simulink model "robot005"  (R2016a)
settings: Solver=FixedStepDiscrete  StartTime=0.0  StopTime=inf  FixedStep=0.001  RelTol=1e-3
libraries: SIA_Robot_Toolbox x9
settings Model: SimulationMode=external  Creator=Administrator  LastModifiedBy=HP
settings OptimizationCC: OptimizeModelRefInitCode=on  LifeSpan=Inf
settings RTWCC: SystemTargetFile=linux_ert_target.tlc  GenCodeOnly=on  MakeCommand=make_rtw CC=gcc  TemplateMakefile=linux_ert_target.tmf  Description=Linux Embedded Real-Time target  RetainRTWFile=on
settings CodeAppCC: ForceParamTrailComments=on  IgnoreCustomStorageClasses=off  OperatorAnnotations=on  SimulinkDataObjDesc=on  SFDataObjDesc=on  MATLABFcnDesc=on  InsertBlockDesc=on  MATLABSourceComments=on
settings STFCustomTargetCC: CombineOutputUpdateFcns=on  ERTCustomFileBanners=on  SupportNonInlinedSFcns=off  MATLABClassNameForMDSCustomization=Simulink.SoftwareTarget.ERTCustomization  GRTInterface=off  SystemTargetFile=linux_ert_target.tlc
settings ERTTargetCC: ParMdlRefBuildCompliant=off  CompOptLevelCompliant=off  ConcurrentExecutionCompliant=off  SupportContinuousTime=on  ModelStepFunctionPrototypeControlCompliant=off  CPPClassGenCompliant=off  UseToolchainInfoCompliant=off  ExtMode=on  ExtModeMexArgs='192.168.0.99' 1 17725  ERTSrcFileBannerTemplate=linux_ert_target_code_template.cgt  ERTHdrFileBannerTemplate=linux_ert_target_code_template.cgt  ERTDataSrcFileTemplate=linux_ert_target_code_template.cgt  ERTDataHdrFileTemplate=linux_ert_target_code_template.cgt  ERTCustomFileTemplate=linux_ert_target_generate_main.tlc
settings SimscapeCC: SimscapeNormalizeSystem=off

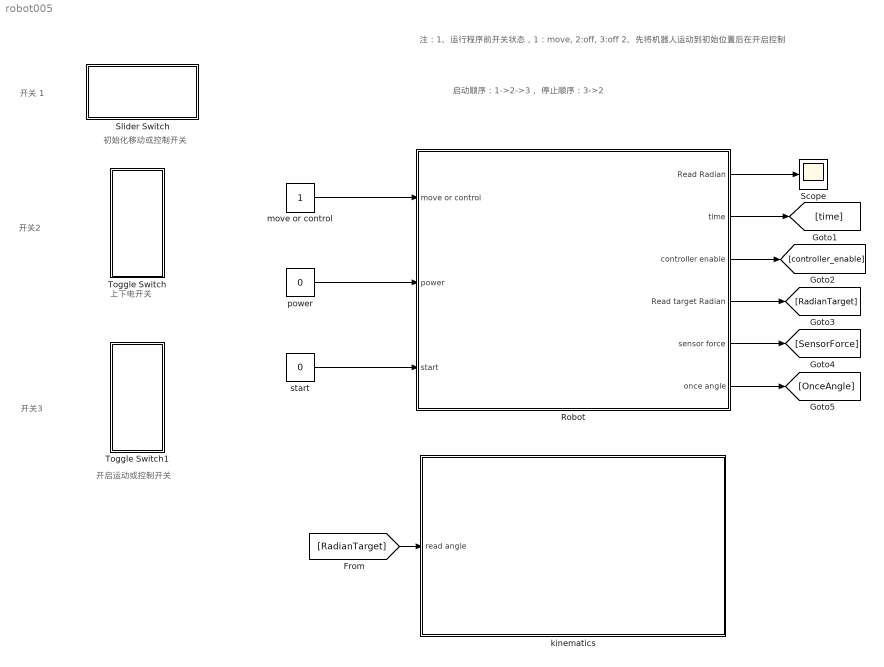
== system robot005 ==
  note: 启动顺序：1->2->3，
      | 停止顺序：3->2
  note: 开关 1
  note: 注：1、运行程序前开关状态，1：move, 2:off, 3:off
      | 2、先将机器人运动到初始位置后在开启控制
  note: 开启运动或控制开关
  note: 上下电开关
  note: 初始化移动或控制开关
  note: 开关2
  note: 开关3
  Robot : Subsystem  mask(模块说明){move_joint=[1 0.6 0 0 1 0]}
      mask prompts: move_joint "move_joint(rad)"
      mask help: 不需要更改该模块内部程序。
  Scope : Scope
  Slider Switch : Subsystem  DialogController=hmiCreateDDGDialog  IsWebBlock=on  mask(MWDashboardBlock){webBlockId=e487defa-cf66-408f-93df-043974d5a550, webBlockType=sliderswitch, ShowInLibBrowser=on, ShowInitialText=on, HMISrcModelName=robot005_2016a}
      mask prompts: webBlockId "WebBlock Id"; webBlockType "WebBlock Type"; HMISrcModelName "Source Model"
      mask help: Set on/off value to tune parameters or variables.
      mask Help: helpview([docroot '/mapfiles/simulink.map'], 'hmi_switch')
      mask Display:
      | if strcmp(get_param(bdroot(gcb),'BlockDiagramType'),'library')
      |  image([(matlabroot) '/toolbox/simulink/hmi/icons/SliderSwitch.png'])
      | end
  Toggle Switch : Subsystem  DialogController=hmiCreateDDGDialog  IsWebBlock=on  mask(MWDashboardBlock){webBlockId=df158d09-57bd-48b0-a65e-f3d7cce1d0b3, webBlockType=toggleswitch, ShowInLibBrowser=on, ShowInitialText=on, HMISrcModelName=robot005_2016a}
      mask prompts: webBlockId "WebBlock Id"; webBlockType "WebBlock Type"; HMISrcModelName "Source Model"
      mask help: Set on/off value to tune parameters or variables.
      mask Help: helpview([docroot '/mapfiles/simulink.map'], 'hmi_switch')
      mask Display:
      | if strcmp(get_param(bdroot(gcb),'BlockDiagramType'),'library')
      |  image([(matlabroot) '/toolbox/simulink/hmi/icons/ToggleSwitch.png'])
      | end
  Toggle Switch1 : Subsystem  DialogController=hmiCreateDDGDialog  IsWebBlock=on  mask(MWDashboardBlock){webBlockId=392d6191-f6a5-4e6d-a801-0994c69ad5e5, webBlockType=toggleswitch, ShowInLibBrowser=on, ShowInitialText=on, HMISrcModelName=robot005_2016a}
      mask prompts: webBlockId "WebBlock Id"; webBlockType "WebBlock Type"; HMISrcModelName "Source Model"
      mask help: Set on/off value to tune parameters or variables.
      mask Help: helpview([docroot '/mapfiles/simulink.map'], 'hmi_switch')
      mask Display:
      | if strcmp(get_param(bdroot(gcb),'BlockDiagramType'),'library')
      |  image([(matlabroot) '/toolbox/simulink/hmi/icons/ToggleSwitch.png'])
      | end
  kinematics : Subsystem
  move or control : Constant
  power : Constant  Value=0
  start : Constant  Value=0
  wires:
  move or control/1 -> Robot/1(move or control)
  power/1 -> Robot/2(power)
  Robot/1(Read Radian) -> Scope/1
  Robot/2(time) -> [time]
  Robot/3(controller enable) -> [controller_enable]
  Robot/4(Read target Radian) -> [RadianTarget]
  Robot/5(sensor force) -> [SensorForce]
  Robot/6(once angle) -> [OnceAngle]
  start/1 -> Robot/3(start)
  [RadianTarget] -> kinematics/1(read angle)

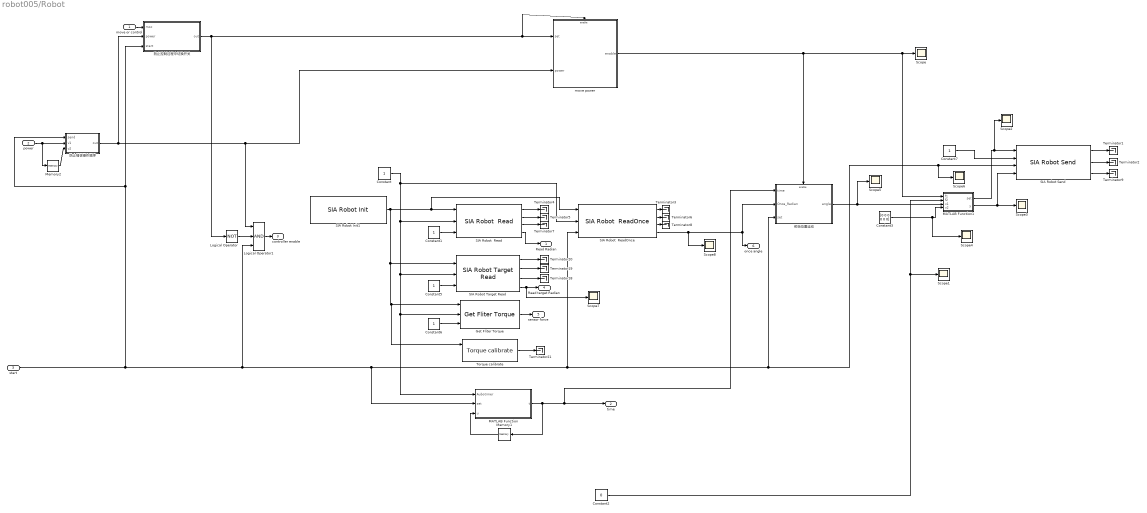
== system robot005/Robot ==
  move or control : Inport
  power : Inport  Port=2
  start : Inport  Port=3
  " Torque calibrate" : SIA_Robot_Toolbox/Sensor/ Torque calibrate
  Constant{,1,5..7} (5 alike) : Constant
  Constant2 : Constant  Value=0
  Constant3 : Constant  Value=[0 0 0 0 0 0]
  Get Fliter Torque : SIA_Robot_Toolbox/Sensor/Get Fliter Torque  p_buf_num_sensor=20
  Logical Operator : Logic  Operator=NOT  AllPortsSameDT=off  OutDataTypeStr=boolean
  Logical Operator1 : Logic  Inputs=3  AllPortsSameDT=off  OutDataTypeStr=boolean
  MATLAB Function : MATLAB Function  TreatAsAtomicUnit=on
  MATLAB Function1 : MATLAB Function  TreatAsAtomicUnit=on
  Memory1 : Memory
  Memory2 : Memory
  SIA Robot  Read : SIA_Robot_Toolbox/Robot Interface/SIA Robot  Read  g_Axisnum=6
  SIA Robot  ReadOnce : SIA_Robot_Toolbox/Robot Interface/SIA Robot  ReadOnce  g_Axisnum=6
  SIA Robot Init1 : SIA_Robot_Toolbox/Robot System Tool/SIA Robot Init  p_AUBO=on
  SIA Robot Send : SIA_Robot_Toolbox/Robot Interface/SIA Robot Send  g_Axisnum=6
  SIA Robot Target Read : SIA_Robot_Toolbox/Robot Interface/SIA Robot Target Read
  Scope{,1..8} (9 alike) : Scope
  Terminator{1..9,18..21} (13 alike) : Terminator
  move power : Subsystem
  初始位置运动 : Subsystem
  防止控制过程中切换开关 : MATLAB Function  TreatAsAtomicUnit=on
  防止错误操作顺序 : MATLAB Function  TreatAsAtomicUnit=on
  Read Radian : Outport
  time : Outport  Port=2
  controller enable : Outport  Port=3
  Read target Radian : Outport  Port=4
  sensor force : Outport  Port=5
  once angle : Outport  Port=6
  wires:
  Constant/1 -> SIA Robot  ReadOnce/2, SIA Robot  Read/2, SIA Robot Target Read/2, MATLAB Function/1(Aubotimer), Get Fliter Torque/2
  SIA Robot Init1/1 -> " Torque calibrate"/1, Get Fliter Torque/1, SIA Robot Target Read/1, SIA Robot  ReadOnce/1, SIA Robot  Read/1
  Constant1/1 -> SIA Robot  Read/3
  Memory1/1 -> MATLAB Function/3(u)
  SIA Robot Send/1 -> Terminator1/1
  SIA Robot Send/2 -> Terminator2/1
  SIA Robot  ReadOnce/1 -> Terminator3/1
  SIA Robot  Read/4 -> Read Radian/1
  SIA Robot  ReadOnce/4 -> Scope8/1, 初始位置运动/2(Once_Radian), once angle/1
  MATLAB Function/1(t) -> 初始位置运动/1(time), time/1, Memory1/1
  start/1 -> 防止控制过程中切换开关/3(start), 防止错误操作顺序/1(send), Logical Operator1/3, MATLAB Function/2(set), SIA Robot  ReadOnce/3, 初始位置运动/3(set), Scope6/1, SIA Robot Send/3
  SIA Robot  Read/1 -> Terminator4/1
  SIA Robot  Read/2 -> Terminator5/1
  SIA Robot  ReadOnce/2 -> Terminator6/1
  SIA Robot  Read/3 -> Terminator7/1
  SIA Robot  ReadOnce/3 -> Terminator8/1
  SIA Robot Send/3 -> Terminator9/1
  初始位置运动/1(angle) -> MATLAB Function1/3(v1), Scope5/1
  防止错误操作顺序/1(out) -> 防止控制过程中切换开关/2(power), Logical Operator1/1, move power/2(power)
  防止控制过程中切换开关/1(out) -> Logical Operator/1, move power/Enable, move power/1(set)
  move or control/1 -> 防止控制过程中切换开关/1(moc)
  Memory2/1 -> 防止错误操作顺序/3(v2)
  power/1 -> Memory2/1, 防止错误操作顺序/2(v1)
  Logical Operator1/1 -> controller enable/1
  Logical Operator/1 -> Logical Operator1/2
  Constant5/1 -> SIA Robot Target Read/3
  SIA Robot Target Read/4 -> Scope7/1, Read target Radian/1
  SIA Robot Target Read/3 -> Terminator18/1
  SIA Robot Target Read/2 -> Terminator19/1
  SIA Robot Target Read/1 -> Terminator20/1
  Constant6/1 -> Get Fliter Torque/3
  Get Fliter Torque/1 -> sensor force/1
  " Torque calibrate"/1 -> Terminator21/1
  Constant7/1 -> SIA Robot Send/2
  MATLAB Function1/1(set) -> Scope2/1, SIA Robot Send/1
  Constant3/1 -> Scope4/1, MATLAB Function1/4(v2)
  MATLAB Function1/2(y) -> Scope3/1, SIA Robot Send/4
  move power/1(enable) -> 初始位置运动/Enable, MATLAB Function1/1(f1), Scope/1
  Constant2/1 -> MATLAB Function1/2(f2), Scope1/1

== system robot005/Slider Switch ==

== system robot005/Toggle Switch ==

== system robot005/Toggle Switch1 ==

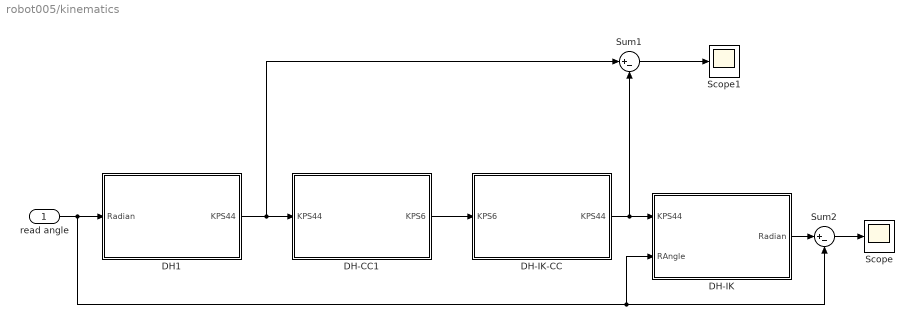
== system robot005/kinematics ==
  read angle : Inport
  DH-CC1 : MATLAB Function  TreatAsAtomicUnit=on
  DH-IK : MATLAB Function  TreatAsAtomicUnit=on
  DH-IK-CC : MATLAB Function  TreatAsAtomicUnit=on
  DH1 : MATLAB Function  TreatAsAtomicUnit=on
  Scope : Scope
  Scope1 : Scope
  Sum1 : Sum  Inputs=|+-
  Sum2 : Sum  Inputs=|+-
  wires:
  DH1/1(KPS44) -> DH-CC1/1(KPS44), Sum1/1
  read angle/1 -> DH1/1(Radian), DH-IK/2(RAngle), Sum2/2
  DH-CC1/1(KPS6) -> DH-IK-CC/1(KPS6)
  DH-IK-CC/1(KPS44) -> DH-IK/1(KPS44), Sum1/2
  DH-IK/1(Radian) -> Sum2/1
  Sum2/1 -> Scope/1
  Sum1/1 -> Scope1/1

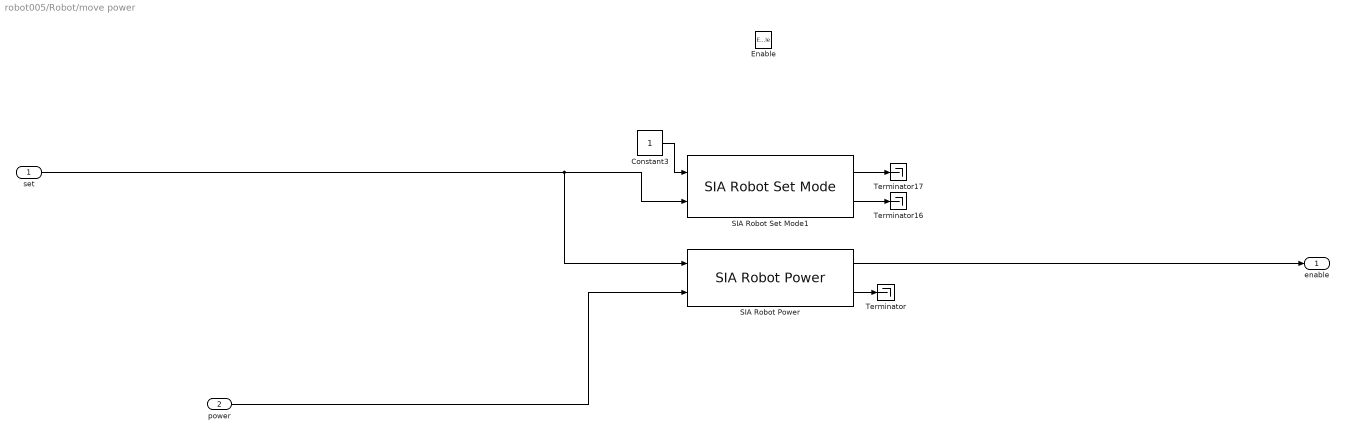
== system robot005/Robot/move power ==
  set : Inport
  power : Inport  Port=2
  Enable : EnablePort
  Constant3 : Constant
  SIA Robot Power : SIA_Robot_Toolbox/Robot System Tool/SIA Robot Power
  SIA Robot Set Mode1 : SIA_Robot_Toolbox/Robot Interface/SIA Robot Set Mode  Axis_1=off  Axis_2=off  Axis_3=off  Axis_4=off  Axis_5=off  Axis_6=off
      link override S-Function Builder: Parameters=Axis_1,Axis_2,Axis_3,Axis_4,Axis_5,Axis_6
  Terminator : Terminator
  Terminator16 : Terminator
  Terminator17 : Terminator
  enable : Outport
  wires:
  power/1 -> SIA Robot Power/2
  set/1 -> SIA Robot Power/1, SIA Robot Set Mode1/2
  SIA Robot Power/2 -> Terminator/1
  Constant3/1 -> SIA Robot Set Mode1/1
  SIA Robot Power/1 -> enable/1
  SIA Robot Set Mode1/2 -> Terminator16/1
  SIA Robot Set Mode1/1 -> Terminator17/1

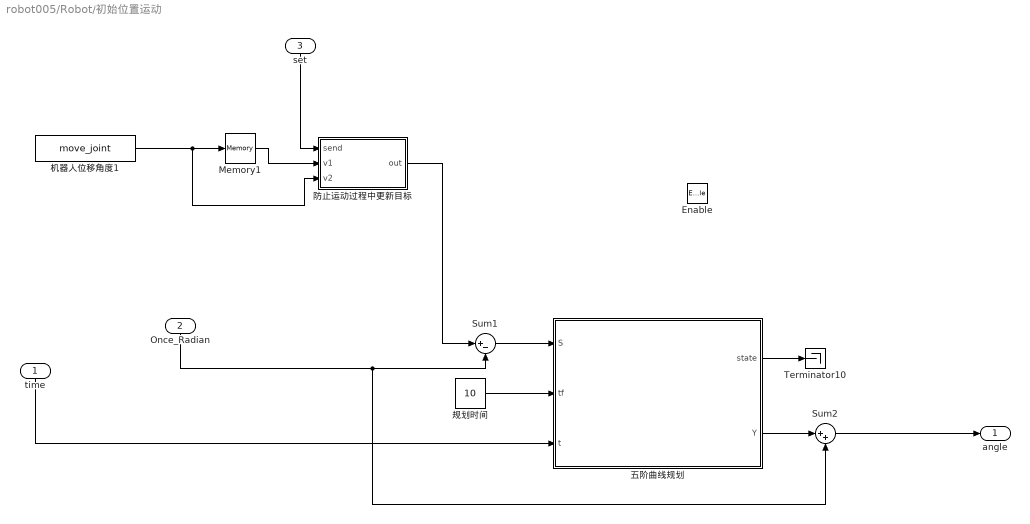
== system robot005/Robot/初始位置运动 ==
  time : Inport
  Once_Radian : Inport  Port=2
  set : Inport  Port=3
  Enable : EnablePort
  Memory1 : Memory  X0=[0 0 0 0 0 0]
  Sum1 : Sum  Inputs=|+-
  Sum2 : Sum  Inputs=|++
  Terminator10 : Terminator
  五阶曲线规划 : Subsystem
  机器人位移角度1 : Constant  Value=move_joint
  规划时间 : Constant  Value=10
  防止运动过程中更新目标 : MATLAB Function  TreatAsAtomicUnit=on
  angle : Outport
  wires:
  五阶曲线规划/2(Y) -> Sum2/1
  Once_Radian/1 -> Sum2/2, Sum1/2
  规划时间/1 -> 五阶曲线规划/2(tf)
  Sum1/1 -> 五阶曲线规划/1(S)
  五阶曲线规划/1(state) -> Terminator10/1
  time/1 -> 五阶曲线规划/3(t)
  Sum2/1 -> angle/1
  set/1 -> 防止运动过程中更新目标/1(send)
  防止运动过程中更新目标/1(out) -> Sum1/1
  机器人位移角度1/1 -> 防止运动过程中更新目标/3(v2), Memory1/1
  Memory1/1 -> 防止运动过程中更新目标/2(v1)

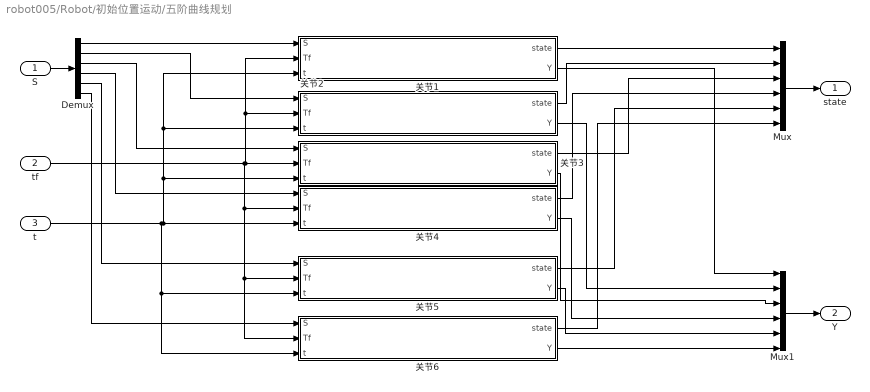
== system robot005/Robot/初始位置运动/五阶曲线规划 ==
  S : Inport
  tf : Inport  Port=2
  t : Inport  Port=3
  Demux : Demux  Outputs=6
  Mux : Mux  Inputs=6
  Mux1 : Mux  Inputs=6
  关节1 : Subsystem
  关节2 : Subsystem
  关节3 : Subsystem
  关节4 : Subsystem
  关节5 : Subsystem
  关节6 : Subsystem
  state : Outport
  Y : Outport  Port=2
  wires:
  关节6/1(state) -> Mux/6
  关节5/1(state) -> Mux/5
  Mux/1 -> state/1
  关节6/2(Y) -> Mux1/6
  关节5/2(Y) -> Mux1/5
  关节4/2(Y) -> Mux1/4
  关节3/2(Y) -> Mux1/3
  关节2/2(Y) -> Mux1/2
  Mux1/1 -> Y/1
  Demux/1 -> 关节1/1(S)
  S/1 -> Demux/1
  关节4/1(state) -> Mux/4
  关节2/1(state) -> Mux/2
  关节3/1(state) -> Mux/3
  关节1/1(state) -> Mux/1
  关节1/2(Y) -> Mux1/1
  Demux/2 -> 关节2/1(S)
  Demux/3 -> 关节3/1(S)
  Demux/4 -> 关节4/1(S)
  Demux/5 -> 关节5/1(S)
  Demux/6 -> 关节6/1(S)
  tf/1 -> 关节6/2(Tf), 关节5/2(Tf), 关节4/2(Tf), 关节3/2(Tf), 关节1/2(Tf), 关节2/2(Tf)
  t/1 -> 关节6/3(t), 关节5/3(t), 关节4/3(t), 关节3/3(t), 关节1/3(t), 关节2/3(t)

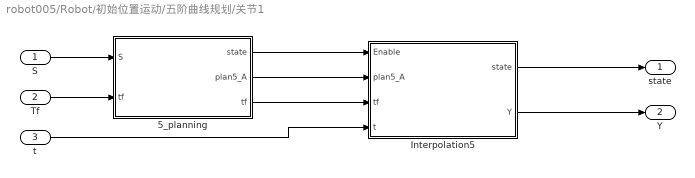
== system robot005/Robot/初始位置运动/五阶曲线规划/关节1 ==
  S : Inport
  Tf : Inport  Port=2
  t : Inport  Port=3
  5_planning : MATLAB Function  TreatAsAtomicUnit=on  mask{g_vs=0, g_ve=0, g_as=0, g_ae=0}
      mask prompts: g_vs "初始速度"; g_ve "末速度"; g_as "初始加速度"; g_ae "末加速度"
  Interpolation5 : MATLAB Function  TreatAsAtomicUnit=on
  state : Outport
  Y : Outport  Port=2
  wires:
  Interpolation5/1(state) -> state/1
  Interpolation5/2(Y) -> Y/1
  Tf/1 -> 5_planning/2("tf ")
  5_planning/3(tf) -> Interpolation5/3(tf)
  5_planning/2(plan5_A) -> Interpolation5/2(plan5_A)
  5_planning/1(state) -> Interpolation5/1(Enable)
  S/1 -> 5_planning/1(S)
  t/1 -> Interpolation5/4(t)

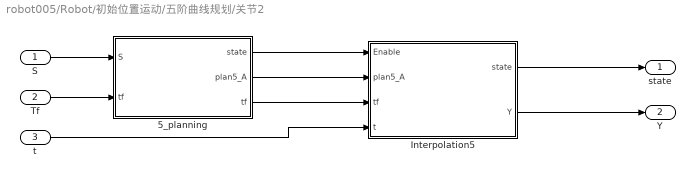
== system robot005/Robot/初始位置运动/五阶曲线规划/关节2 ==
  S : Inport
  Tf : Inport  Port=2
  t : Inport  Port=3
  5_planning : MATLAB Function  TreatAsAtomicUnit=on  mask{g_vs=0, g_ve=0, g_as=0, g_ae=0}
      mask prompts: g_vs "初始速度"; g_ve "末速度"; g_as "初始加速度"; g_ae "末加速度"
  Interpolation5 : MATLAB Function  TreatAsAtomicUnit=on
  state : Outport
  Y : Outport  Port=2
  wires:
  t/1 -> Interpolation5/4(t)
  S/1 -> 5_planning/1(S)
  5_planning/1(state) -> Interpolation5/1(Enable)
  5_planning/2(plan5_A) -> Interpolation5/2(plan5_A)
  5_planning/3(tf) -> Interpolation5/3(tf)
  Tf/1 -> 5_planning/2("tf ")
  Interpolation5/2(Y) -> Y/1
  Interpolation5/1(state) -> state/1

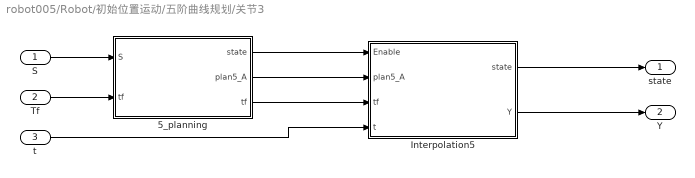
== system robot005/Robot/初始位置运动/五阶曲线规划/关节3 ==
  S : Inport
  Tf : Inport  Port=2
  t : Inport  Port=3
  5_planning : MATLAB Function  TreatAsAtomicUnit=on  mask{g_vs=0, g_ve=0, g_as=0, g_ae=0}
      mask prompts: g_vs "初始速度"; g_ve "末速度"; g_as "初始加速度"; g_ae "末加速度"
  Interpolation5 : MATLAB Function  TreatAsAtomicUnit=on
  state : Outport
  Y : Outport  Port=2
  wires:
  Interpolation5/1(state) -> state/1
  Interpolation5/2(Y) -> Y/1
  Tf/1 -> 5_planning/2("tf ")
  5_planning/3(tf) -> Interpolation5/3(tf)
  5_planning/2(plan5_A) -> Interpolation5/2(plan5_A)
  5_planning/1(state) -> Interpolation5/1(Enable)
  S/1 -> 5_planning/1(S)
  t/1 -> Interpolation5/4(t)

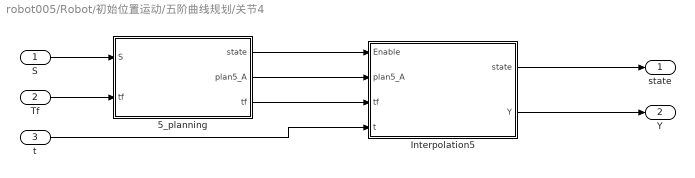
== system robot005/Robot/初始位置运动/五阶曲线规划/关节4 ==
  S : Inport
  Tf : Inport  Port=2
  t : Inport  Port=3
  5_planning : MATLAB Function  TreatAsAtomicUnit=on  mask{g_vs=0, g_ve=0, g_as=0, g_ae=0}
      mask prompts: g_vs "初始速度"; g_ve "末速度"; g_as "初始加速度"; g_ae "末加速度"
  Interpolation5 : MATLAB Function  TreatAsAtomicUnit=on
  state : Outport
  Y : Outport  Port=2
  wires:
  t/1 -> Interpolation5/4(t)
  S/1 -> 5_planning/1(S)
  5_planning/1(state) -> Interpolation5/1(Enable)
  5_planning/2(plan5_A) -> Interpolation5/2(plan5_A)
  5_planning/3(tf) -> Interpolation5/3(tf)
  Tf/1 -> 5_planning/2("tf ")
  Interpolation5/2(Y) -> Y/1
  Interpolation5/1(state) -> state/1

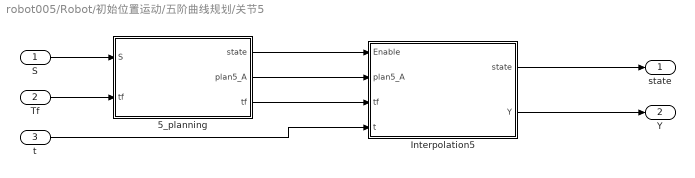
== system robot005/Robot/初始位置运动/五阶曲线规划/关节5 ==
  S : Inport
  Tf : Inport  Port=2
  t : Inport  Port=3
  5_planning : MATLAB Function  TreatAsAtomicUnit=on  mask{g_vs=0, g_ve=0, g_as=0, g_ae=0}
      mask prompts: g_vs "初始速度"; g_ve "末速度"; g_as "初始加速度"; g_ae "末加速度"
  Interpolation5 : MATLAB Function  TreatAsAtomicUnit=on
  state : Outport
  Y : Outport  Port=2
  wires:
  Interpolation5/1(state) -> state/1
  Interpolation5/2(Y) -> Y/1
  Tf/1 -> 5_planning/2("tf ")
  5_planning/3(tf) -> Interpolation5/3(tf)
  5_planning/2(plan5_A) -> Interpolation5/2(plan5_A)
  5_planning/1(state) -> Interpolation5/1(Enable)
  S/1 -> 5_planning/1(S)
  t/1 -> Interpolation5/4(t)

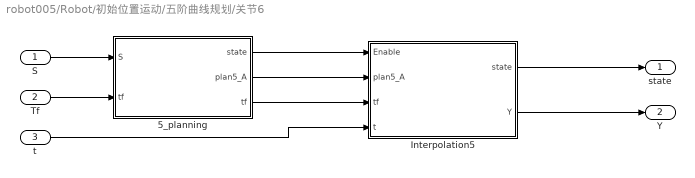
== system robot005/Robot/初始位置运动/五阶曲线规划/关节6 ==
  S : Inport
  Tf : Inport  Port=2
  t : Inport  Port=3
  5_planning : MATLAB Function  TreatAsAtomicUnit=on  mask{g_vs=0, g_ve=0, g_as=0, g_ae=0}
      mask prompts: g_vs "初始速度"; g_ve "末速度"; g_as "初始加速度"; g_ae "末加速度"
  Interpolation5 : MATLAB Function  TreatAsAtomicUnit=on
  state : Outport
  Y : Outport  Port=2
  wires:
  t/1 -> Interpolation5/4(t)
  S/1 -> 5_planning/1(S)
  5_planning/1(state) -> Interpolation5/1(Enable)
  5_planning/2(plan5_A) -> Interpolation5/2(plan5_A)
  5_planning/3(tf) -> Interpolation5/3(tf)
  Tf/1 -> 5_planning/2("tf ")
  Interpolation5/2(Y) -> Y/1
  Interpolation5/1(state) -> state/1

== matlab function robot005/Robot/MATLAB Function ==
  data: Aubotimer input; set input; u input; t output
  function t = Aubotime(Aubotimer,set,u)
%#codegen
persistent flag;
if isempty(flag)
flag = 0;
end
if(set == 1)   
    t = u+0.001;
else
    t = 0;
end

== matlab function robot005/Robot/初始位置运动/五阶曲线规划/关节2/5_planning ==
  data: S input; tf input; state output; plan5_A output; g_vs parameter; g_ve parameter; tf output; g_as parameter; g_ae parameter
function [state, plan5_A,tf] =planning5( S,tf,g_vs, g_ve, g_as, g_ae)
% 五次多项式算法主程序
% vs初始速度m/min,ve末速度m/min
% as初始加速度，ae末加速度
% S总位移m,tf为规划时间
% 基础插补规划函数
% 五次多项式速度规划
    a=zeros(1,6);
    a(1) = 0 ;
    a(2) = g_vs ;
    a(3) = g_as/2;
    a(4) = (20*S - (8*g_ve + 12 * g_vs )*tf - (3*g_as - g_ae)*tf^2)/(2*tf^3);
    a(5) = (-30*S + (14*g_ve + 16 * g_vs )*tf + (3*g_as - 2*g_ae)*tf^2)/(2*tf^4);
    a(6) = (12*S - 6*(g_ve + g_vs )*tf + (g_ae - g_as)*tf^2)/(2*tf^5);
    
    state1 = 1;
    state = state1;
    plan5_A = a;
    tf =tf ;
end

== matlab function robot005/Robot/初始位置运动/五阶曲线规划/关节1/5_planning ==
  data: S input; tf input; state output; plan5_A output; g_vs parameter; g_ve parameter; tf output; g_as parameter; g_ae parameter
function [state, plan5_A,tf] =planning5( S,tf,g_vs, g_ve, g_as, g_ae)
% 五次多项式算法主程序
% vs初始速度m/min,ve末速度m/min
% as初始加速度，ae末加速度
% S总位移m,tf为规划时间
% 基础插补规划函数
% 五次多项式速度规划
    a=zeros(1,6);
    a(1) = 0 ;
    a(2) = g_vs ;
    a(3) = g_as/2;
    a(4) = (20*S - (8*g_ve + 12 * g_vs )*tf - (3*g_as - g_ae)*tf^2)/(2*tf^3);
    a(5) = (-30*S + (14*g_ve + 16 * g_vs )*tf + (3*g_as - 2*g_ae)*tf^2)/(2*tf^4);
    a(6) = (12*S - 6*(g_ve + g_vs )*tf + (g_ae - g_as)*tf^2)/(2*tf^5);
    
    state1 = 1;
    state = state1;
    plan5_A = a;
    tf =tf ;
end

== matlab function robot005/Robot/初始位置运动/五阶曲线规划/关节2/Interpolation5 ==
  data: state output; Enable input; Y output; plan5_A input; tf input; t input
function [state, Y]  = Interpolate5(Enable,plan5_A,tf,t)
%% input
a0 = plan5_A(1);
a1 = plan5_A(2);
a2 = plan5_A(3);
a3 = plan5_A(4);
a4 = plan5_A(5);
a5 = plan5_A(6);
Y = 0;
%% output
if Enable == 1
    if t <=tf
    Y = a0 + a1*t + a2*t^2 + a3*t^3 + a4*t^4 + a5*t^5; 
    state =1;
    else
    Y = a0 + a1*tf + a2*tf^2 + a3*tf^3 + a4*tf^4 + a5*tf^5;
    state = 1;
    end
else 
    Y = 0;
    state = 0;
end
end

== matlab function robot005/Robot/初始位置运动/五阶曲线规划/关节3/5_planning ==
  data: S input; tf input; state output; plan5_A output; g_vs parameter; g_ve parameter; tf output; g_as parameter; g_ae parameter
function [state, plan5_A,tf] =planning5( S,tf,g_vs, g_ve, g_as, g_ae)
% 五次多项式算法主程序
% vs初始速度m/min,ve末速度m/min
% as初始加速度，ae末加速度
% S总位移m,tf为规划时间
% 基础插补规划函数
% 五次多项式速度规划
    a=zeros(1,6);
    a(1) = 0 ;
    a(2) = g_vs ;
    a(3) = g_as/2;
    a(4) = (20*S - (8*g_ve + 12 * g_vs )*tf - (3*g_as - g_ae)*tf^2)/(2*tf^3);
    a(5) = (-30*S + (14*g_ve + 16 * g_vs )*tf + (3*g_as - 2*g_ae)*tf^2)/(2*tf^4);
    a(6) = (12*S - 6*(g_ve + g_vs )*tf + (g_ae - g_as)*tf^2)/(2*tf^5);
    
    state1 = 1;
    state = state1;
    plan5_A = a;
    tf =tf ;
end

== matlab function robot005/Robot/初始位置运动/五阶曲线规划/关节3/Interpolation5 ==
  data: state output; Enable input; Y output; plan5_A input; tf input; t input
function [state, Y]  = Interpolate5(Enable,plan5_A,tf,t)
%% input
a0 = plan5_A(1);
a1 = plan5_A(2);
a2 = plan5_A(3);
a3 = plan5_A(4);
a4 = plan5_A(5);
a5 = plan5_A(6);
Y = 0;
%% output
if Enable == 1
    if t <=tf
    Y = a0 + a1*t + a2*t^2 + a3*t^3 + a4*t^4 + a5*t^5; 
    state =1;
    else
    Y = a0 + a1*tf + a2*tf^2 + a3*tf^3 + a4*tf^4 + a5*tf^5;
    state = 1;
    end
else 
    Y = 0;
    state = 0;
end
end

== matlab function robot005/Robot/初始位置运动/五阶曲线规划/关节4/5_planning ==
  data: S input; tf input; state output; plan5_A output; g_vs parameter; g_ve parameter; tf output; g_as parameter; g_ae parameter
function [state, plan5_A,tf] =planning5( S,tf,g_vs, g_ve, g_as, g_ae)
% 五次多项式算法主程序
% vs初始速度m/min,ve末速度m/min
% as初始加速度，ae末加速度
% S总位移m,tf为规划时间
% 基础插补规划函数
% 五次多项式速度规划
    a=zeros(1,6);
    a(1) = 0 ;
    a(2) = g_vs ;
    a(3) = g_as/2;
    a(4) = (20*S - (8*g_ve + 12 * g_vs )*tf - (3*g_as - g_ae)*tf^2)/(2*tf^3);
    a(5) = (-30*S + (14*g_ve + 16 * g_vs )*tf + (3*g_as - 2*g_ae)*tf^2)/(2*tf^4);
    a(6) = (12*S - 6*(g_ve + g_vs )*tf + (g_ae - g_as)*tf^2)/(2*tf^5);
    
    state1 = 1;
    state = state1;
    plan5_A = a;
    tf =tf ;
end

== matlab function robot005/Robot/初始位置运动/五阶曲线规划/关节4/Interpolation5 ==
  data: state output; Enable input; Y output; plan5_A input; tf input; t input
function [state, Y]  = Interpolate5(Enable,plan5_A,tf,t)
%% input
a0 = plan5_A(1);
a1 = plan5_A(2);
a2 = plan5_A(3);
a3 = plan5_A(4);
a4 = plan5_A(5);
a5 = plan5_A(6);
Y = 0;
%% output
if Enable == 1
    if t <=tf
    Y = a0 + a1*t + a2*t^2 + a3*t^3 + a4*t^4 + a5*t^5; 
    state =1;
    else
    Y = a0 + a1*tf + a2*tf^2 + a3*tf^3 + a4*tf^4 + a5*tf^5;
    state = 1;
    end
else 
    Y = 0;
    state = 0;
end
end

== matlab function robot005/Robot/初始位置运动/五阶曲线规划/关节5/5_planning ==
  data: S input; tf input; state output; plan5_A output; g_vs parameter; g_ve parameter; tf output; g_as parameter; g_ae parameter
function [state, plan5_A,tf] =planning5( S,tf,g_vs, g_ve, g_as, g_ae)
% 五次多项式算法主程序
% vs初始速度m/min,ve末速度m/min
% as初始加速度，ae末加速度
% S总位移m,tf为规划时间
% 基础插补规划函数
% 五次多项式速度规划
    a=zeros(1,6);
    a(1) = 0 ;
    a(2) = g_vs ;
    a(3) = g_as/2;
    a(4) = (20*S - (8*g_ve + 12 * g_vs )*tf - (3*g_as - g_ae)*tf^2)/(2*tf^3);
    a(5) = (-30*S + (14*g_ve + 16 * g_vs )*tf + (3*g_as - 2*g_ae)*tf^2)/(2*tf^4);
    a(6) = (12*S - 6*(g_ve + g_vs )*tf + (g_ae - g_as)*tf^2)/(2*tf^5);
    
    state1 = 1;
    state = state1;
    plan5_A = a;
    tf =tf ;
end

== matlab function robot005/Robot/初始位置运动/五阶曲线规划/关节5/Interpolation5 ==
  data: state output; Enable input; Y output; plan5_A input; tf input; t input
function [state, Y]  = Interpolate5(Enable,plan5_A,tf,t)
%% input
a0 = plan5_A(1);
a1 = plan5_A(2);
a2 = plan5_A(3);
a3 = plan5_A(4);
a4 = plan5_A(5);
a5 = plan5_A(6);
Y = 0;
%% output
if Enable == 1
    if t <=tf
    Y = a0 + a1*t + a2*t^2 + a3*t^3 + a4*t^4 + a5*t^5; 
    state =1;
    else
    Y = a0 + a1*tf + a2*tf^2 + a3*tf^3 + a4*tf^4 + a5*tf^5;
    state = 1;
    end
else 
    Y = 0;
    state = 0;
end
end

== matlab function robot005/Robot/初始位置运动/五阶曲线规划/关节6/5_planning ==
  data: S input; tf input; state output; plan5_A output; g_vs parameter; g_ve parameter; tf output; g_as parameter; g_ae parameter
function [state, plan5_A,tf] =planning5( S,tf,g_vs, g_ve, g_as, g_ae)
% 五次多项式算法主程序
% vs初始速度m/min,ve末速度m/min
% as初始加速度，ae末加速度
% S总位移m,tf为规划时间
% 基础插补规划函数
% 五次多项式速度规划
    a=zeros(1,6);
    a(1) = 0 ;
    a(2) = g_vs ;
    a(3) = g_as/2;
    a(4) = (20*S - (8*g_ve + 12 * g_vs )*tf - (3*g_as - g_ae)*tf^2)/(2*tf^3);
    a(5) = (-30*S + (14*g_ve + 16 * g_vs )*tf + (3*g_as - 2*g_ae)*tf^2)/(2*tf^4);
    a(6) = (12*S - 6*(g_ve + g_vs )*tf + (g_ae - g_as)*tf^2)/(2*tf^5);
    
    state1 = 1;
    state = state1;
    plan5_A = a;
    tf =tf ;
end

== matlab function robot005/Robot/初始位置运动/五阶曲线规划/关节6/Interpolation5 ==
  data: state output; Enable input; Y output; plan5_A input; tf input; t input
function [state, Y]  = Interpolate5(Enable,plan5_A,tf,t)
%% input
a0 = plan5_A(1);
a1 = plan5_A(2);
a2 = plan5_A(3);
a3 = plan5_A(4);
a4 = plan5_A(5);
a5 = plan5_A(6);
Y = 0;
%% output
if Enable == 1
    if t <=tf
    Y = a0 + a1*t + a2*t^2 + a3*t^3 + a4*t^4 + a5*t^5; 
    state =1;
    else
    Y = a0 + a1*tf + a2*tf^2 + a3*tf^3 + a4*tf^4 + a5*tf^5;
    state = 1;
    end
else 
    Y = 0;
    state = 0;
end
end

== matlab function robot005/Robot/防止控制过程中切换开关 ==
  data: moc input; power input; start input; out output
  function out = move_control_deal(moc,power,start)
%#codegen
persistent flag;
if isempty(flag)
flag = 0;
end
persistent flag1;
if isempty(flag1)
flag1 = 0;
end

if ((0==power)&&(0==start))
   out=moc;
   flag1=moc;
else
    if (0==flag)
      flag1=moc;
    end
    out=flag1;
end

    flag=1;

  end

== matlab function robot005/Robot/初始位置运动/五阶曲线规划/关节1/Interpolation5 ==
  data: state output; Enable input; Y output; plan5_A input; tf input; t input
function [state, Y]  = Interpolate5(Enable,plan5_A,tf,t)
%% input
a0 = plan5_A(1);
a1 = plan5_A(2);
a2 = plan5_A(3);
a3 = plan5_A(4);
a4 = plan5_A(5);
a5 = plan5_A(6);
Y = 0;
%% output
if Enable == 1
    if t <=tf
    Y = a0 + a1*t + a2*t^2 + a3*t^3 + a4*t^4 + a5*t^5; 
    state =1;
    else
    Y = a0 + a1*tf + a2*tf^2 + a3*tf^3 + a4*tf^4 + a5*tf^5;
    state = 1;
    end
else 
    Y = 0;
    state = 0;
end
end

== matlab function robot005/Robot/防止错误操作顺序 ==
  data: send input; v1 input; out output; v2 input
function out  = update(send,v1,v2)
persistent flag;
if isempty(flag)
flag = 0;
end

persistent out_;
if isempty(out_)
out_ = 0;
end

if (0==v1)
    out=v1;
    flag=0;
else
    if ((v1>v2)&&(1==send))
       out=v2;
       out_=0;
       flag=1;
    else
        if (1==flag)
           out=0;
        else
           out=v1;
        end
    
    end
end
end

== matlab function robot005/kinematics/DH-IK ==
  data: KPS44 input; Radian output; RAngle input
function Radian  = IK(KPS44,RAngle)
%% DH parameter(单位：mm)
Radian = zeros(1,6);
%XB4
d1=342;a1=40;a2=275;a3=25;d4=280;dt=73;d3=0;

Tbase = [1 0 0 0;
        0 1 0 0;
        0 0 1 d1;
        0 0 0 1];
Ttool = [1 0 0 0;
        0 1 0 0;
        0 0 1 dt;
        0 0 0 1];
inv_Tbase = inv(Tbase);
inv_Ttool = inv(Ttool);
%% input 
%逆运动学,参数u为4*4变换矩阵(单位：mm)
%Q_为当前机器人角度（单位:rad）
%返回值new_Q为计算出的关节角度（单位：rad）
%%QQ为8*6矩阵，存放八组解
R44 = inv_Tbase*KPS44*inv_Ttool;
theta1 = RAngle(1);
theta2 = RAngle(2);
theta3 = RAngle(3);
theta4 = RAngle(4);
theta5 = RAngle(5);
theta6 = RAngle(6);
offset2 = -pi/2; offset3 = 0;
Q_=[theta1;theta2+offset2;theta3+offset3;theta4;theta5;theta6];
%% 由实际姿态矩阵转换成建模姿态矩阵    
r=[R44(1,1) R44(1,2) R44(1,3);
   R44(2,1) R44(2,2) R44(2,3);
   R44(3,1) R44(3,2) R44(3,3)];
%% 位置
x=R44(1,4);y=R44(2,4);z=R44(3,4);
nx=R44(1,1);ny=R44(2,1);nz=R44(3,1);
ox=R44(1,2);oy=R44(2,2);oz=R44(3,2);
ax=R44(1,3);ay=R44(2,3);az=R44(3,3);
%% parameter
Q1=zeros(1,2);
Q3=zeros(1,4);
Q2=zeros(2,2);
Q23=zeros(2,2);
Q4=zeros(2,2);
Q5=zeros(2,2);
Q6=zeros(2,2);

Qmin = [0 0 0 0 0 0];
Qmax = [0 0 0 0 0 0];
QQ = zeros(8,6);
%new_Q = zeros(1,6);
bz =zeros(1,8);
Min =zeros(1,8);

%%求取角度1




%%求取角度3








%%求取角度2、4、5、6



















%四组解变成八组            









%-----------角度上下限设定-----------
%Q_=[theta1;theta2-pi/2;theta3;theta4+pi/2;theta5;theta6];
Qmin(1)=-170*(pi/180);Qmax(1)=170*(pi/180);
Qmin(2)=-80*(pi/180);Qmax(2)=144*(pi/180);
Qmin(3)=-194*(pi/180);Qmax(3)=54*(pi/180);
Qmin(4)=-170*(pi/180);Qmax(4)=170*(pi/180);
Qmin(5)=-119*(pi/180);Qmax(5)=119*(pi/180);
Qmin(6)=-360*(pi/180);Qmax(6)=360*(pi/180);
%------------逆解完善-----------
for m=1:8
   for n=1:6
      if (QQ(m,n)<Qmin(n)) 
         QQ(m,n)=QQ(m,n)+2*pi;
      end
      if (QQ(m,n)>Qmax(n))
          QQ(m,n)=QQ(m,n)-2*pi;
      end    
      %防止角度跳跃
      if abs(QQ(m,n)-Q_(n)>pi) %#ok<ELARLOG>
          if (QQ(m,n)>=0)
              QQ(m,n)=QQ(m,n)-2*pi;
          else
              QQ(m,n)=QQ(m,n)+2*pi;
          end
      end  
   end   
end
 %--------筛选可行解
   for h=1:8    
       if ((QQ(h,1)>=Qmin(1))&&(QQ(h,1)<=Qmax(1)))&&((QQ(h,2)>=Qmin(2))&&(QQ(h,2)<=Qmax(2)))&&((QQ(h,3)>=Qmin(3))&&(QQ(h,3)<=Qmax(3)))&&((QQ(h,4)>=Qmin(4))&&(QQ(h,4)<=Qmax(4)))&&((QQ(h,5)>=Qmin(5))&&(QQ(h,5)<=Qmax(5)))&&((QQ(h,6)>=Qmin(6))&&(QQ(h,6)<=Qmax(6)))
           bz(h)=1;%可行解标志，为1是表示是可行解
           Min(h)=abs(Q_(1)-QQ(h,1))+abs(Q_(2)-QQ(h,2))+abs(Q_(3)-QQ(h,3))+abs(Q_(4)-QQ(h,4))+abs(Q_(5)-QQ(h,5))+abs(Q_(6)-QQ(h,6));%计算对应解的值
       else
           bz(h)=0;
           Min(h)=0;
       end
   end  
%------从可行解中找到最优解











Radian = new_Q;
end

== matlab function robot005/kinematics/DH1 ==
  data: Radian input; KPS44 output
function KPS44  = FK(Radian)

%% input 
theta1 = Radian(1);
theta2 = Radian(2);
theta3 = Radian(3);
theta4 = Radian(4);
theta5 = Radian(5);
theta6 = Radian(6);

%% D-H parameters 
%XB4
 d1=342;a1=40;a2=275;a3=25;d4=280;dt=73;d3=0;



%% output
II = zeros(4,4);

%% T1~T6

     
     
KPS44 = Tbase*II*Ttool;



end

== matlab function robot005/kinematics/DH-IK-CC ==
  data: KPS6 input; KPS44 output
function KPS44  = IK(KPS6)
%% input 
x = KPS6(1);
y = KPS6(2);
z = KPS6(3);
p = KPS6(4);
q = KPS6(5);
r = KPS6(6);
%% output
I= diag(ones(1,4));
%%固定角到齐次变换
sx = sin(p);
cx = cos(p);
sy = sin(q);
cy = cos(q);
sz = sin(r);
cz = cos(r);
KPS44(1,1) =		
KPS44(1,2) =	
KPS44(1,3) =
KPS44(2,1) = 	
KPS44(2,2) = 	
KPS44(2,3) = 
KPS44(3,1) =	
KPS44(3,2) =	
KPS44(3,3) =
KPS44(1,4) = 
KPS44(2,4) =
KPS44(3,4) =
KPS44(4,4) = 

end

== matlab function robot005/kinematics/DH-CC1 ==
  data: KPS44 input; KPS6 output
function KPS6  = FK(KPS44)
%% parameter
rpy = zeros(1,3);
eps = 0.000001;
%% input 

%%output
 
end

== matlab function robot005/Robot/初始位置运动/防止运动过程中更新目标 ==
  data: send input; v1 input; out output; v2 input
function out  = update(send,v1,v2)
v1=reshape(v1,1,6);
v2=reshape(v2,1,6);
persistent flag;
if isempty(flag)
flag = 0;
end

persistent out_;
if isempty(out_)
out_ = zeros(1,6);
end

if (1==send)
    if ((norm(v1-v2)>0.001)||1==flag)
        out=out_;
        flag=1;
    else
        out=v2;
        out_=v2;
    end
else
    out=v2;
    out_=v2;
    flag=0;
end
end

== matlab function robot005/Robot/MATLAB Function1 ==
  data: set output; f1 input; y output; f2 input; v1 input; v2 input
function [set,y] = fcn(f1,f2,v1,v2)
%#codegen
v1=reshape(v1,6,1);
v2=reshape(v2,6,1);
if ((1==f1)||(1==f2))
    set=1;
else
    set=0;
end

if (1==f1)
   y=v1; 
else
    if (1==f2)
       y=v2; 
    else
       y=zeros(6,1); 
    end
end

end
